simulink model "cbuildv1p1"  (R2024b)
settings: Solver=VariableStepAuto  StartTime=0.0  StopTime=2  RelTol=1e-3
model workspace (MAT data in the model file):
  A_busbar = 0.0015
  A_pack = 0.711626248
  C = 400
  C_nominal = 3
  GR = 14.14
  I_max = 157.708978328
  Izz = 76.97
  P = 5
  P_DD = 1
  REGEN_GAIN = 1
  R_e = 0.197
  S = 138
  SW_TV_GAIN = 0.035
  SoC_initial = 1
  TC_CUT = 0.5
  T_amb = 297.15
  Tmax = 21
  W_max = 34
  a = 0.7497
  busbar_CC_area = 0.000108
  busbar_Cp = 237
  busbar_length = 0.032
  busbar_mass = 0.01
  busbar_resistivity = 1.68e-08
  busbar_thermalcontact_resistance = 1
  c_factor = 0.244
  cell_Cp = 1000
  cell_mass = 0.046
  deg_to_rad = 0.0174533
  g = 9.81
  h_busbar = 5
  h_pack = 5
  kappa_thresh = 0.12
  l = 1.53
  mpersec_to_kph = 3.6
  rackdisp_to_steerangle = 1.29615626969
  rad_to_deg = 57.2958
  rpm_to_radpers = 0.10472
libraries: Solver_SF x1
settings Model: Creator=account  LastModifiedBy=kara.28

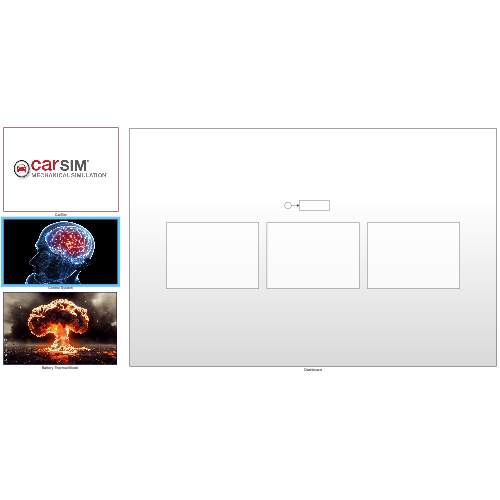
[thumbnail: Simulink's stored preview of the top-level diagram]
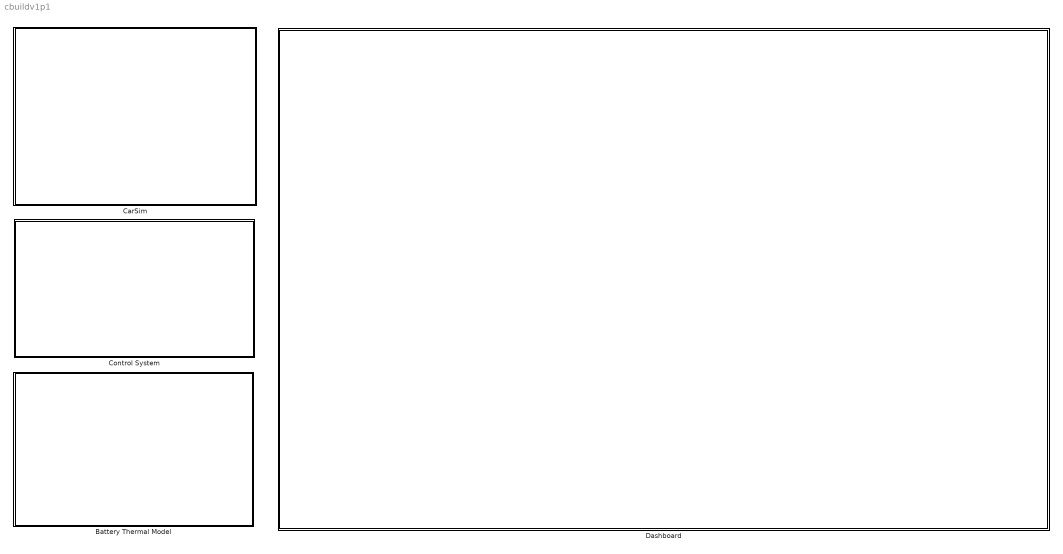
== system cbuildv1p1 ==
  Battery Thermal Model : Subsystem
      mask Display: image('battery.jpg');
  CarSim : Subsystem
      mask Display: image('carsimlogo.jpg');
  Control System : Subsystem
      mask Display: image('controller.jpg');
  Dashboard : Subsystem

== system cbuildv1p1/Battery Thermal Model ==
  Battery Cells : Subsystem
  Busbars : Subsystem

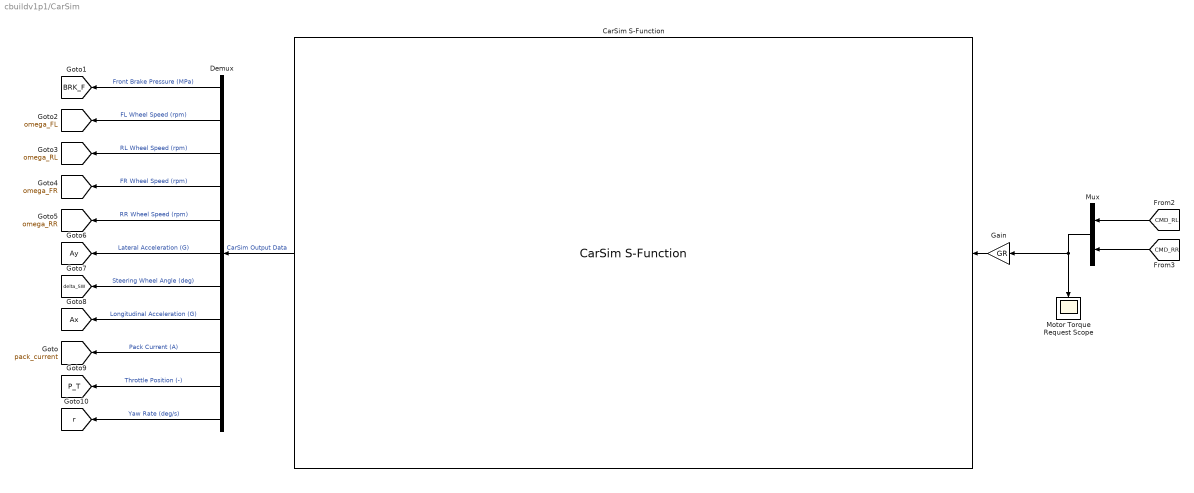
== system cbuildv1p1/CarSim ==
  CarSim S-Function : Solver_SF/CarSim S-Function  Priority=1  SIMFILE=simfile.sim  Run_RTs=off  vs_state_ind=Run  StopMode_ind=Vehicle Model
  Demux : Demux  Outputs=11
  Gain : Gain  Gain=GR
  Motor Torque Request Scope : Scope
  Mux : Mux  Inputs=2
  tag scope: Ax=global, Ay=global, BRK_F=global, P_T=global, delta_SW=global, omega_FL=global, omega_FR=global, omega_RL=global, omega_RR=global, pack_current=global, r=global
  wires:
  Demux/5 -> [omega_RR]  "RR Wheel Speed (rpm)"
  Demux/10 -> [P_T]  "Throttle Position (-)"
  Demux/8 -> [Ax]  "Longitudinal Acceleration (G)"
  Demux/4 -> [omega_FR]  "FR Wheel Speed (rpm)"
  Demux/2 -> [omega_FL]  "FL Wheel Speed (rpm)"
  CarSim S-Function/1 -> Demux/1  "CarSim Output Data"
  Demux/7 -> [delta_SW]  "Steering Wheel Angle (deg)"
  [CMD_RR] -> Mux/2
  [CMD_RL] -> Mux/1
  Demux/9 -> [pack_current]  "Pack Current (A)"
  Demux/3 -> [omega_RL]  "RL Wheel Speed (rpm)"
  Demux/1 -> [BRK_F]  "Front Brake Pressure (MPa)"
  Demux/6 -> [Ay]  "Lateral Acceleration (G)"
  Gain/1 -> CarSim S-Function/1
  Mux/1 -> Gain/1, Motor Torque Request Scope/1
  Demux/11 -> [r]  "Yaw Rate (deg/s)"

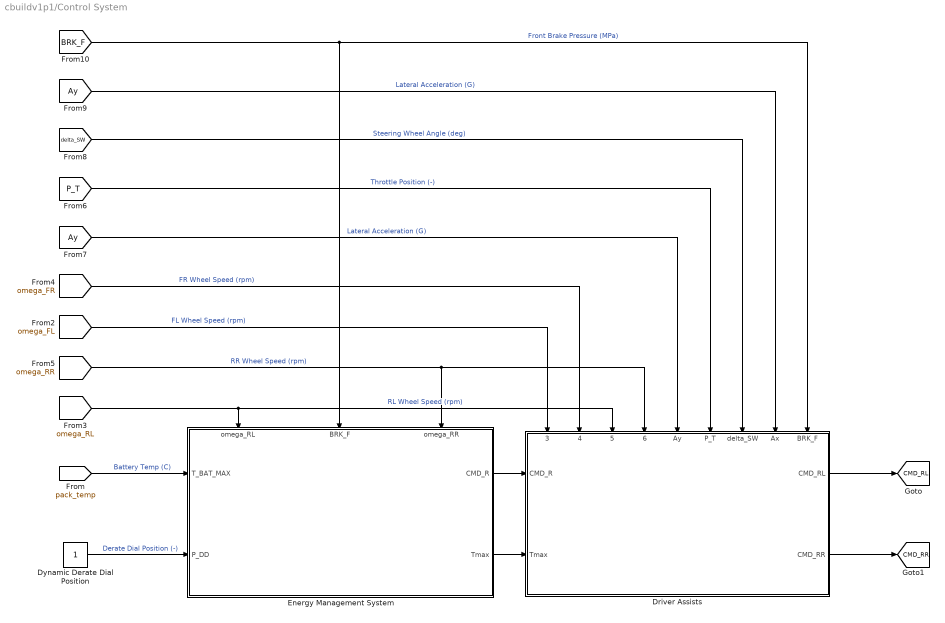
== system cbuildv1p1/Control System ==
  Driver Assists : Subsystem
      settings: PortSchema="{\"entries\":[{\"content\":{\"sides\":[{\"content\":{\"connectorIds\":[\"In1\",\"In2\"]},\"type\":\"ConnectorPlacement.EquallySpacedRectSide\",\"uuid\":\"c30f5bbb-5f7b-4b8f-a220-579b9cc0865f\"},{\"content\":{\"connectorIds\":[\"Out1\",\"Out2\"],\"side\":\"RIGHT\"},\"type\":\"ConnectorPlacement.EquallySpacedRectSide\",\"uuid\":\"8399a92e-19c3-49c4-801c-f7e7f76799cf\"},{\"content\":{\"connectorIds\":[\"In3\",\"In4\",\"In5\",\"In6\",\"In7\",\"In8\",\"In9\",\"In10\",\"In11\"],\"side\":\"TOP\"},\"type\":\"ConnectorPlacement.EquallySpacedRectSide\",\"uuid\":\"19d8375b-8353-4f23-adee-fcd0b0fbd4ef\"}]},\"type\":\"ConnectorPlacement.EquallySpacedConnector\",\"uuid\":\"53834b5a-6686-42bc-a078-9cae71bfd001\"}],\"packageUris\":[\"http://schema.mathworks.com/mf0/Connector/R2020b\"],\"version\":\"1.0\"}"
  Dynamic Derate Dial Position : Constant
  Energy Management System : Subsystem
      settings: PortSchema="{\"entries\":[{\"content\":{\"sides\":[{\"content\":{\"connectorIds\":[\"In1\",\"In2\"]},\"type\":\"ConnectorPlacement.EquallySpacedRectSide\",\"uuid\":\"89c92abe-ca77-4c48-ba79-1fd8447b36ee\"},{\"content\":{\"connectorIds\":[\"Out1\",\"Out2\"],\"side\":\"RIGHT\"},\"type\":\"ConnectorPlacement.EquallySpacedRectSide\",\"uuid\":\"4a58accb-bbe3-490f-b1ea-5257f75ab2ba\"},{\"content\":{\"connectorIds\":[\"In3\",\"In4\",\"In5\"],\"side\":\"TOP\"},\"type\":\"ConnectorPlacement.EquallySpacedRectSide\",\"uuid\":\"b5e96e52-1098-4ccd-9740-b2b10d8cf6b3\"}]},\"type\":\"ConnectorPlacement.EquallySpacedConnector\",\"uuid\":\"06c6d35a-fc7b-4382-b862-8bbe65743431\"}],\"packageUris\":[\"http://schema.mathworks.com/mf0/Connector/R2020b\"],\"version\":\"1.0\"}"
  tag scope: CMD_RL=global, CMD_RR=global
  wires:
  Energy Management System/1(CMD_R) -> Driver Assists/1(CMD_R)
  Energy Management System/2(Tmax) -> Driver Assists/2(Tmax)
  Driver Assists/1(CMD_RL) -> [CMD_RL]
  Driver Assists/2(CMD_RR) -> [CMD_RR]
  [pack_temp] -> Energy Management System/1(T_BAT_MAX)  "Battery Temp (C)"
  Dynamic Derate Dial Position/1 -> Energy Management System/2(P_DD)  "Derate Dial Position (-)"
  [omega_RR] -> Driver Assists/6(omega_RR), Energy Management System/5(omega_RR)  "RR Wheel Speed (rpm)"
  [omega_FR] -> Driver Assists/4(omega_FR)  "FR Wheel Speed (rpm)"
  [omega_RL] -> Driver Assists/5(omega_RL), Energy Management System/3(omega_RL)  "RL Wheel Speed (rpm)"
  [omega_FL] -> Driver Assists/3(omega_FL)  "FL Wheel Speed (rpm)"
  [Ay] -> Driver Assists/7(Ay)  "Lateral Acceleration (G)"
  [P_T] -> Driver Assists/8(P_T)  "Throttle Position (-)"
  [delta_SW] -> Driver Assists/9(delta_SW)  "Steering Wheel Angle (deg)"
  [Ay] -> Driver Assists/10(Ax)  "Lateral Acceleration (G)"
  [BRK_F] -> Energy Management System/4(BRK_F), Driver Assists/11(BRK_F)  "Front Brake Pressure (MPa)"

== system cbuildv1p1/Dashboard ==
  Battery Info : Subsystem
  Clock1 : Clock
  Controls Info : Subsystem
  General Info : Subsystem
  Simulation Time : Display
  wires:
  Clock1/1 -> Simulation Time/1

== system cbuildv1p1/Battery Thermal Model/Battery Cells ==
  Battery Heat : Subsystem
      settings: PortSchema="{\"entries\":[{\"content\":{\"sides\":[{\"content\":{\"connectorIds\":[\"In1\",\"Out1\",\"In2\",\"In3\"]},\"type\":\"ConnectorPlacement.EquallySpacedRectSide\",\"uuid\":\"0f7c0562-63f7-413a-9c65-7d5d0f23ac53\"},{\"content\":{\"side\":\"RIGHT\"},\"type\":\"ConnectorPlacement.EquallySpacedRectSide\",\"uuid\":\"6856fc4a-e601-47fb-aafe-3183d6398fa2\"},{\"content\":{\"side\":\"TOP\"},\"type\":\"ConnectorPlacement.EquallySpacedRectSide\",\"uuid\":\"93500152-ab0c-4e86-a765-8796b82b9cd6\"}]},\"type\":\"ConnectorPlacement.EquallySpacedConnector\",\"uuid\":\"8bef09a8-0835-4033-ba4e-3f5f6277d0ac\"}],\"packageUris\":[\"http://schema.mathworks.com/mf0/Connector/R2020b\"],\"version\":\"1.0\"}"
  Battery Heat Generation : Subsystem
  Busbar - Segment Heat Flow : Subsystem
      settings: PortSchema="{\"entries\":[{\"content\":{\"sides\":[{\"content\":{},\"type\":\"ConnectorPlacement.EquallySpacedRectSide\",\"uuid\":\"839c7b7c-3d90-4543-803d-828e2cd8ee3e\"},{\"content\":{\"connectorIds\":[\"In1\",\"Out1\"],\"side\":\"RIGHT\"},\"type\":\"ConnectorPlacement.EquallySpacedRectSide\",\"uuid\":\"e3492608-3f40-473c-8392-0c925b682872\"},{\"content\":{\"side\":\"TOP\"},\"type\":\"ConnectorPlacement.EquallySpacedRectSide\",\"uuid\":\"8e15337c-e61d-491c-b508-620217c9bb60\"}]},\"type\":\"ConnectorPlacement.EquallySpacedConnector\",\"uuid\":\"03d3ec16-7a24-4203-9805-446eb586226e\"}],\"packageUris\":[\"http://schema.mathworks.com/mf0/Connector/R2020b\"],\"version\":\"1.0\"}"
  Heat Loss : Subsystem
      settings: PortSchema="{\"entries\":[{\"content\":{\"sides\":[{\"content\":{},\"type\":\"ConnectorPlacement.EquallySpacedRectSide\",\"uuid\":\"cd11f8f0-ebc0-4dda-8c98-00f5919de41a\"},{\"content\":{\"connectorIds\":[\"In1\",\"Out1\"],\"side\":\"RIGHT\"},\"type\":\"ConnectorPlacement.EquallySpacedRectSide\",\"uuid\":\"2a68a9a1-bd97-4a17-8a8b-1aa98e9bd9a8\"},{\"content\":{\"side\":\"TOP\"},\"type\":\"ConnectorPlacement.EquallySpacedRectSide\",\"uuid\":\"debcc510-941b-4448-a371-f67c84c59f32\"}]},\"type\":\"ConnectorPlacement.EquallySpacedConnector\",\"uuid\":\"91559e46-754b-48b4-ac3e-ab135f9add0a\"}],\"packageUris\":[\"http://schema.mathworks.com/mf0/Connector/R2020b\"],\"version\":\"1.0\"}"
  Pack Voltage : Subsystem
  wires:
  Battery Heat/1(Pack Temp (K)) -> Busbar - Segment Heat Flow/1(Segment Temp (K)), Heat Loss/1(Pack Temp (K))
  Battery Heat Generation/1(Cell Heat Generation Rate) -> Battery Heat/1(Battery Heat Generation)
  Heat Loss/1(Pack Heat Loss Rate) -> Battery Heat/2(Battery Heat Loss)
  Busbar - Segment Heat Flow/1(Busbar - Segment Heat Flow (W)) -> Battery Heat/3(Busbar - Segment Heat Flow (W))

== system cbuildv1p1/Battery Thermal Model/Busbars ==
  Ambient Heat Loss : Subsystem
      settings: PortSchema="{\"entries\":[{\"content\":{\"sides\":[{\"content\":{},\"type\":\"ConnectorPlacement.EquallySpacedRectSide\",\"uuid\":\"cd11f8f0-ebc0-4dda-8c98-00f5919de41a\"},{\"content\":{\"connectorIds\":[\"In1\",\"Out1\"],\"side\":\"RIGHT\"},\"type\":\"ConnectorPlacement.EquallySpacedRectSide\",\"uuid\":\"2a68a9a1-bd97-4a17-8a8b-1aa98e9bd9a8\"},{\"content\":{\"side\":\"TOP\"},\"type\":\"ConnectorPlacement.EquallySpacedRectSide\",\"uuid\":\"debcc510-941b-4448-a371-f67c84c59f32\"}]},\"type\":\"ConnectorPlacement.EquallySpacedConnector\",\"uuid\":\"91559e46-754b-48b4-ac3e-ab135f9add0a\"}],\"packageUris\":[\"http://schema.mathworks.com/mf0/Connector/R2020b\"],\"version\":\"1.0\"}"
  Busbar - Segment Heat Flow : Subsystem
      settings: PortSchema="{\"entries\":[{\"content\":{\"sides\":[{\"content\":{},\"type\":\"ConnectorPlacement.EquallySpacedRectSide\",\"uuid\":\"839c7b7c-3d90-4543-803d-828e2cd8ee3e\"},{\"content\":{\"connectorIds\":[\"In1\",\"Out1\"],\"side\":\"RIGHT\"},\"type\":\"ConnectorPlacement.EquallySpacedRectSide\",\"uuid\":\"e3492608-3f40-473c-8392-0c925b682872\"},{\"content\":{\"side\":\"TOP\"},\"type\":\"ConnectorPlacement.EquallySpacedRectSide\",\"uuid\":\"8e15337c-e61d-491c-b508-620217c9bb60\"}]},\"type\":\"ConnectorPlacement.EquallySpacedConnector\",\"uuid\":\"03d3ec16-7a24-4203-9805-446eb586226e\"}],\"packageUris\":[\"http://schema.mathworks.com/mf0/Connector/R2020b\"],\"version\":\"1.0\"}"
  Busbar Heat : Subsystem
      settings: PortSchema="{\"entries\":[{\"content\":{\"sides\":[{\"content\":{\"connectorIds\":[\"In1\",\"Out1\",\"In2\",\"In3\"]},\"type\":\"ConnectorPlacement.EquallySpacedRectSide\",\"uuid\":\"0f7c0562-63f7-413a-9c65-7d5d0f23ac53\"},{\"content\":{\"side\":\"RIGHT\"},\"type\":\"ConnectorPlacement.EquallySpacedRectSide\",\"uuid\":\"6856fc4a-e601-47fb-aafe-3183d6398fa2\"},{\"content\":{\"side\":\"TOP\"},\"type\":\"ConnectorPlacement.EquallySpacedRectSide\",\"uuid\":\"93500152-ab0c-4e86-a765-8796b82b9cd6\"}]},\"type\":\"ConnectorPlacement.EquallySpacedConnector\",\"uuid\":\"8bef09a8-0835-4033-ba4e-3f5f6277d0ac\"}],\"packageUris\":[\"http://schema.mathworks.com/mf0/Connector/R2020b\"],\"version\":\"1.0\"}"
  Resistance Heat Generation : Subsystem
  wires:
  Busbar Heat/1(Busbar Temp (K)) -> Busbar - Segment Heat Flow/1(Busbar Temp (K)), Ambient Heat Loss/1(Busbar Temp (K))
  Resistance Heat Generation/1(Busbar Heat Generation Rate) -> Busbar Heat/1(Busbar Heat Generation)
  Ambient Heat Loss/1(Busbar Heat Loss Rate) -> Busbar Heat/2(Busbar Heat Loss)
  Busbar - Segment Heat Flow/1(Busbar - Segment Heat Flow (W)) -> Busbar Heat/3(Busbar - Segment Heat Flow (W))

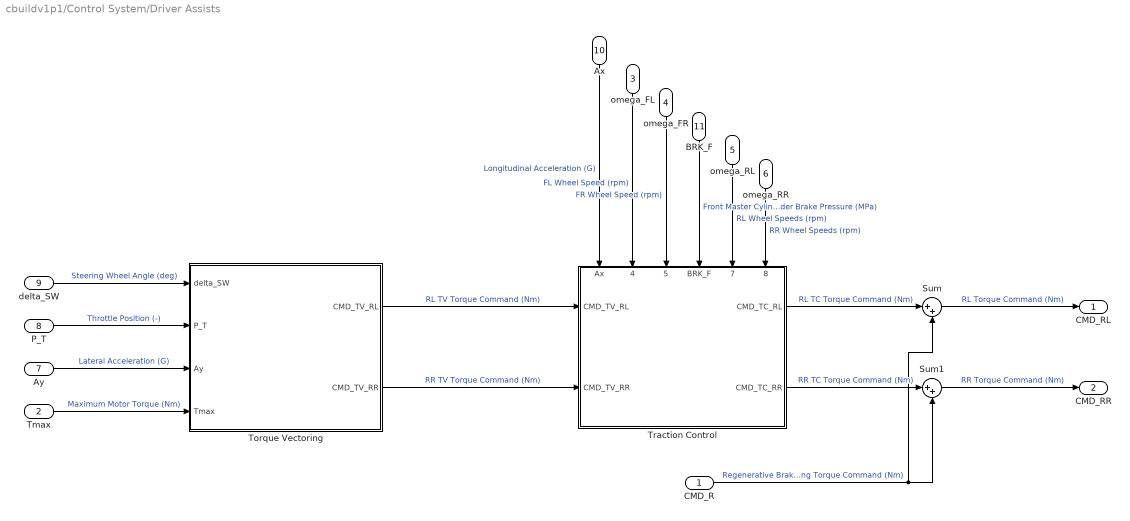
== system cbuildv1p1/Control System/Driver Assists ==
  CMD_R : Inport
  Tmax : Inport  Port=2
  omega_FL : Inport  Port=3
  omega_FR : Inport  Port=4
  omega_RL : Inport  Port=5
  omega_RR : Inport  Port=6
  Ay : Inport  Port=7
  P_T : Inport  Port=8
  delta_SW : Inport  Port=9
  Ax : Inport  Port=10
  BRK_F : Inport  Port=11
  Sum : Sum  Inputs=|++
  Sum1 : Sum  Inputs=|++
  Torque Vectoring : Subsystem
  Traction Control : Subsystem
      settings: PortSchema="{\"entries\":[{\"content\":{\"sides\":[{\"content\":{\"connectorIds\":[\"In1\",\"In2\"]},\"type\":\"ConnectorPlacement.EquallySpacedRectSide\",\"uuid\":\"d61c18bd-9535-4dda-869d-17effaf93de7\"},{\"content\":{\"connectorIds\":[\"Out1\",\"Out2\"],\"side\":\"RIGHT\"},\"type\":\"ConnectorPlacement.EquallySpacedRectSide\",\"uuid\":\"01ce504d-a060-4358-8411-664eedaba102\"},{\"content\":{\"connectorIds\":[\"In3\",\"In4\",\"In5\",\"In6\",\"In7\",\"In8\"],\"side\":\"TOP\"},\"type\":\"ConnectorPlacement.EquallySpacedRectSide\",\"uuid\":\"26eb6c05-86e8-47d0-a1b5-f53131bb5e60\"}]},\"type\":\"ConnectorPlacement.EquallySpacedConnector\",\"uuid\":\"a0cd41b8-03b3-4f62-a25e-73ac641935b2\"}],\"packageUris\":[\"http://schema.mathworks.com/mf0/Connector/R2020b\"],\"version\":\"1.0\"}"
  CMD_RL : Outport
  CMD_RR : Outport  Port=2
  wires:
  Torque Vectoring/2(CMD_TV_RR) -> Traction Control/2(CMD_TV_RR)  "RR TV Torque Command (Nm)"
  delta_SW/1 -> Torque Vectoring/1(delta_SW)  "Steering Wheel Angle (deg)"
  P_T/1 -> Torque Vectoring/2(P_T)  "Throttle Position (-)"
  Ay/1 -> Torque Vectoring/3(Ay)  "Lateral Acceleration (G)"
  Tmax/1 -> Torque Vectoring/4(Tmax)  "Maximum Motor Torque (Nm)"
  Sum/1 -> CMD_RL/1  "RL Torque Command (Nm)"
  Sum1/1 -> CMD_RR/1  "RR Torque Command (Nm)"
  CMD_R/1 -> Sum/2, Sum1/2  "Regenerative Braking Torque Command (Nm)"
  Ax/1 -> Traction Control/3(Ax)  "Longitudinal Acceleration (G)"
  omega_FL/1 -> Traction Control/4(omega_FL)  "FL Wheel Speed (rpm)"
  omega_FR/1 -> Traction Control/5(omega_FR)  "FR Wheel Speed (rpm)"
  BRK_F/1 -> Traction Control/6(BRK_F)  "Front Master Cylinder Brake Pressure (MPa)"
  omega_RL/1 -> Traction Control/7(omega_RL)  "RL Wheel Speeds (rpm)"
  omega_RR/1 -> Traction Control/8(omega_RR)  "RR Wheel Speeds (rpm)"
  Torque Vectoring/1(CMD_TV_RL) -> Traction Control/1(CMD_TV_RL)  "RL TV Torque Command (Nm)"
  Traction Control/1(CMD_TC_RL) -> Sum/1  "RL TC Torque Command (Nm)"
  Traction Control/2(CMD_TC_RR) -> Sum1/1  "RR TC Torque Command (Nm)"

== system cbuildv1p1/Control System/Energy Management System ==
  T_BAT_MAX : Inport
  P_DD : Inport  Port=2
  omega_RL : Inport  Port=3
  BRK_F : Inport  Port=4
  omega_RR : Inport  Port=5
  Dynamic Derate : Subsystem
  Regenerative Braking : Subsystem
  CMD_R : Outport
  Tmax : Outport  Port=2
  wires:
  T_BAT_MAX/1 -> Dynamic Derate/1(T_BAT_MAX)  "Maximum Module Temp (C)"
  P_DD/1 -> Dynamic Derate/2(P_DD)  "Dynamic Derate Dial Position (-)"
  BRK_F/1 -> Regenerative Braking/1(BRK_F)  "Front Master Cylinder Pressure (MPa)"
  Dynamic Derate/1(Tmax) -> Tmax/1  "Maximum Motor Torque (Nm)"
  Regenerative Braking/1(CMD_R) -> CMD_R/1  "Regen Brake Torque Command (Nm)"
  omega_RL/1 -> Dynamic Derate/3(omega_RL)  "RL Wheel Speed (rpm)"
  omega_RR/1 -> Dynamic Derate/4(omega_RR)  "RR Wheel Speed (rpm)"

== system cbuildv1p1/Dashboard/Battery Info ==
  Acceleration Scope : DashboardScope  Ymin=-2.5  Ymax=2.5
  Acceleration Scope1 : DashboardScope  Ymin=0  Ymax=60
  Acceleration Scope2 : DashboardScope  Ymin=0  Ymax=1
  Acceleration Scope3 : DashboardScope  Ymin=0  Ymax=1
  Acceleration Scope4 : DashboardScope  Ymin=0  Ymax=500

== system cbuildv1p1/Dashboard/Controls Info ==
  Acceleration Scope : DashboardScope  Ymin=-2.5  Ymax=2.5
  Acceleration Scope1 : DashboardScope  Ymin=-2  Ymax=2
  Acceleration Scope2 : DashboardScope  Ymin=0  Ymax=1
  Acceleration Scope3 : DashboardScope  Ymin=0  Ymax=80
  Acceleration Scope4 : DashboardScope  Ymin=0  Ymax=21
  Lamp : LampBlock  LabelPosition=Hide
  Rotary Switch : RotarySwitchBlock
      settings: Values={{'DD 1', 'DD 2'}, [0 1]}

== system cbuildv1p1/Dashboard/General Info ==
  Acceleration Scope : DashboardScope  Ymin=-2.5  Ymax=2.5
  Acceleration Scope1 : DashboardScope  Ymin=0  Ymax=110
  Acceleration Scope2 : DashboardScope  Ymin=0  Ymax=1
  Acceleration Scope3 : DashboardScope  Ymin=0  Ymax=10
  Acceleration Scope4 : DashboardScope  Ymin=0  Ymax=150

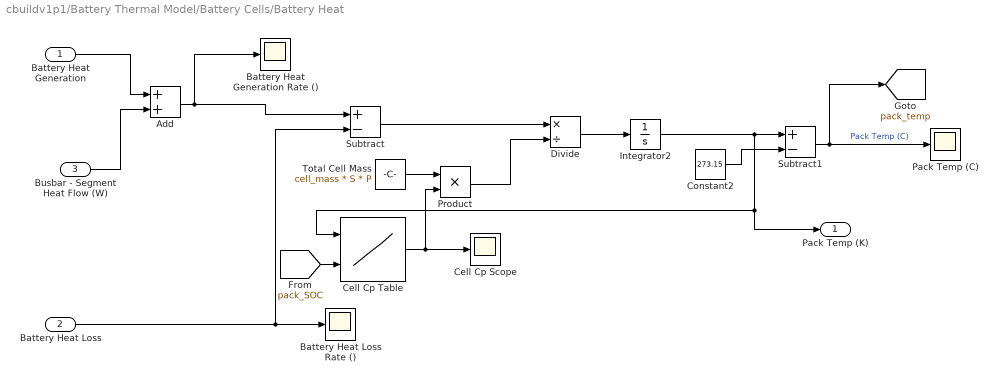
== system cbuildv1p1/Battery Thermal Model/Battery Cells/Battery Heat ==
  Battery Heat Generation : Inport
  Battery Heat Loss : Inport  Port=2
  Busbar - Segment Heat Flow (W) : Inport  Port=3
  Add : Sum
  Battery Heat Generation Rate () : Scope
  Battery Heat Loss Rate () : Scope
  Cell Cp Scope : Scope
  Cell Cp Table : Lookup_n-D  BreakpointsForDimension1=[296.0488;303.3425;312.147;321.5769;330.6423]  BreakpointsForDimension2=[0 0.5 1]  Table=[811.0868 819.6535 830.8545;814.1373 822.704 834.6964;817.9826 826.8129 838.6737000000001;822.2249 831.0552 843.4446;826.7299 835.8239 848.3459]  InterpMethod=Cubic spline  InternalRulePriority=Speed  RndMeth=Simplest
      settings: InputPortMap=u0,u1
  Constant2 : Constant  Value=273.15
  Divide : Product  Inputs=*/
  Integrator2 : Integrator  InitialCondition=T_amb
  Pack Temp (C) : Scope
  Product : Product
  Subtract : Sum  Inputs=+-
  Subtract1 : Sum  Inputs=+-
  Total Cell Mass : Constant  Value=cell_mass * S * P
  Pack Temp (K) : Outport
  tag scope: pack_temp=global
  wires:
  Cell Cp Table/1 -> Product/2, Cell Cp Scope/1
  Constant2/1 -> Subtract1/2
  Divide/1 -> Integrator2/1
  Subtract/1 -> Divide/1
  Integrator2/1 -> Pack Temp (K)/1, Cell Cp Table/1, Subtract1/1
  Subtract1/1 -> [pack_temp], Pack Temp (C)/1  "Pack Temp (C)"
  Total Cell Mass/1 -> Product/1
  Product/1 -> Divide/2
  Battery Heat Loss/1 -> Battery Heat Loss Rate ()/1, Subtract/2
  Battery Heat Generation/1 -> Add/1
  Busbar - Segment Heat Flow (W)/1 -> Add/2
  Add/1 -> Subtract/1, Battery Heat Generation Rate ()/1
  [pack_SOC] -> Cell Cp Table/2

== system cbuildv1p1/Battery Thermal Model/Battery Cells/Battery Heat Generation ==
  Cell Resistance : Subsystem
      settings: PortSchema="{\"entries\":[{\"content\":{\"sides\":[{\"content\":{},\"type\":\"ConnectorPlacement.EquallySpacedRectSide\",\"uuid\":\"1c6ff2a8-2c86-4b92-aa7d-5717a02d6f28\"},{\"content\":{\"connectorIds\":[\"In1\",\"In2\",\"Out1\"],\"side\":\"RIGHT\"},\"type\":\"ConnectorPlacement.EquallySpacedRectSide\",\"uuid\":\"52a4cb2c-e1db-459d-bd0a-206cc3bba6d1\"},{\"content\":{\"side\":\"TOP\"},\"type\":\"ConnectorPlacement.EquallySpacedRectSide\",\"uuid\":\"751bbbd6-abc7-4265-8d68-4aa70d69379f\"}]},\"type\":\"ConnectorPlacement.EquallySpacedConnector\",\"uuid\":\"b8f9630f-0167-4478-8d98-637e13782dcd\"}],\"packageUris\":[\"http://schema.mathworks.com/mf0/Connector/R2020b\"],\"version\":\"1.0\"}"
  Cells in Parallel : Constant  Value=P
  Cells in series : Constant  Value=S
  Current Estimator : Subsystem
  Divide : Product  Inputs=*/
  Pack SoC : Subsystem
      settings: PortSchema="{\"entries\":[{\"content\":{\"sides\":[{\"content\":{},\"type\":\"ConnectorPlacement.EquallySpacedRectSide\",\"uuid\":\"1c6ff2a8-2c86-4b92-aa7d-5717a02d6f28\"},{\"content\":{\"connectorIds\":[\"In1\",\"Out1\"],\"side\":\"RIGHT\"},\"type\":\"ConnectorPlacement.EquallySpacedRectSide\",\"uuid\":\"52a4cb2c-e1db-459d-bd0a-206cc3bba6d1\"},{\"content\":{\"side\":\"TOP\"},\"type\":\"ConnectorPlacement.EquallySpacedRectSide\",\"uuid\":\"751bbbd6-abc7-4265-8d68-4aa70d69379f\"}]},\"type\":\"ConnectorPlacement.EquallySpacedConnector\",\"uuid\":\"b8f9630f-0167-4478-8d98-637e13782dcd\"}],\"packageUris\":[\"http://schema.mathworks.com/mf0/Connector/R2020b\"],\"version\":\"1.0\"}"
  Product : Product
  Product1 : Product
  Product2 : Product
  Square : Math  Operator=square
  Cell Heat Generation Rate : Outport
  wires:
  Cells in series/1 -> Product1/1
  Divide/1 -> Cell Resistance/1(Cell Current  (A)), Square/1  "Cell Current (A)"
  Cell Resistance/1(Cell Resistance (ohms)) -> Product/2  "Cell Resistance (ohms)"
  Square/1 -> Product/1
  Cells in Parallel/1 -> Divide/2, Product1/2
  Product1/1 -> Product2/2
  Product/1 -> Product2/1  "Pack Heat Generation Rate (W)"
  Product2/1 -> Cell Heat Generation Rate/1  "Cell Heat Generation Rate (W)"
  Pack SoC/1(SoC (%)) -> Cell Resistance/2(SoC (%))  "Pack SoC (-)"
  Current Estimator/1(Pack Current (A)) -> Pack SoC/1(Pack Current (A)), Divide/1  "Pack Current (A)"

== system cbuildv1p1/Battery Thermal Model/Battery Cells/Busbar - Segment Heat Flow ==
  Segment Temp (K) : Inport
  Add : Sum
  Constant : Constant  Value=busbar_thermalcontact_resistance
  Constant1 : Constant  Value=273.15
  Divide : Product  Inputs=*/
  Subtract : Sum  Inputs=+-
  Busbar - Segment Heat Flow (W) : Outport
  wires:
  Subtract/1 -> Divide/1  "Temp diff (K)"
  Constant/1 -> Divide/2
  Divide/1 -> Busbar - Segment Heat Flow (W)/1
  [busbar_temp] -> Add/2  "Segment temp (C)"
  Constant1/1 -> Add/1
  Segment Temp (K)/1 -> Subtract/1
  Add/1 -> Subtract/2  "Segment temp (K)"

== system cbuildv1p1/Battery Thermal Model/Battery Cells/Heat Loss ==
  Pack Temp (K) : Inport
  Constant : Constant  Value=h_pack
  Constant1 : Constant  Value=T_amb
  Gain : Gain  Gain=A_pack
  Product : Product
  Scope : Scope
  Subtract : Sum  Inputs=+-
  Pack Heat Loss Rate : Outport
  tag scope: pack_heatloss=global
  wires:
  Constant/1 -> Gain/1
  Subtract/1 -> Product/2, Scope/1
  Gain/1 -> Product/1
  Product/1 -> [pack_heatloss], Pack Heat Loss Rate/1
  Pack Temp (K)/1 -> Subtract/1
  Constant1/1 -> Subtract/2

== system cbuildv1p1/Battery Thermal Model/Battery Cells/Pack Voltage ==
  Gain : Gain  Gain=S
  Lookup with Linear Lagrange Interpolation : Lookup_n-D  NumberOfTableDimensions=1  BreakpointsForDimension1=[0.100961;0.201247;0.30155;0.401865;0.502237;0.602602;0.7029339999999999;0.8032629999999999;0.903617;1]  Table=[3.227877;3.437376;3.537935;3.663634;3.755814;3.835423;3.940172;4.047017;4.097296;4.187904]  InterpMethod=Cubic spline  InternalRulePriority=Speed  RndMeth=Simplest
  tag scope: pack_OCV=global
  wires:
  [pack_SOC] -> Lookup with Linear Lagrange Interpolation/1
  Lookup with Linear Lagrange Interpolation/1 -> Gain/1
  Gain/1 -> [pack_OCV]  "Pack OCV (V)"

== system cbuildv1p1/Battery Thermal Model/Busbars/Ambient Heat Loss ==
  Busbar Temp (K) : Inport
  Ambient temp (K) : Constant  Value=T_amb
  H busbar : Constant  Value=h_busbar
  Product : Product
  Subtract : Sum  Inputs=+-
  busbar area : Gain  Gain=A_busbar
  Busbar Heat Loss Rate : Outport
  tag scope: busbar_heatloss=global
  wires:
  H busbar/1 -> busbar area/1
  Subtract/1 -> Product/2
  busbar area/1 -> Product/1
  Product/1 -> [busbar_heatloss], Busbar Heat Loss Rate/1
  Busbar Temp (K)/1 -> Subtract/1
  Ambient temp (K)/1 -> Subtract/2

== system cbuildv1p1/Battery Thermal Model/Busbars/Busbar - Segment Heat Flow ==
  Busbar Temp (K) : Inport
  Add : Sum
  Constant : Constant  Value=busbar_thermalcontact_resistance
  Constant1 : Constant  Value=273.15
  Divide : Product  Inputs=*/
  Subtract : Sum  Inputs=+-
  Busbar - Segment Heat Flow (W) : Outport
  tag scope: busbar_segment_heatflow=global
  wires:
  Busbar Temp (K)/1 -> Subtract/2
  Subtract/1 -> Divide/1  "Temp diff (K)"
  Constant/1 -> Divide/2
  Divide/1 -> [busbar_segment_heatflow], Busbar - Segment Heat Flow (W)/1
  [pack_temp] -> Add/2  "Segment temp (C)"
  Constant1/1 -> Add/1
  Add/1 -> Subtract/1  "Segment temp (K)"

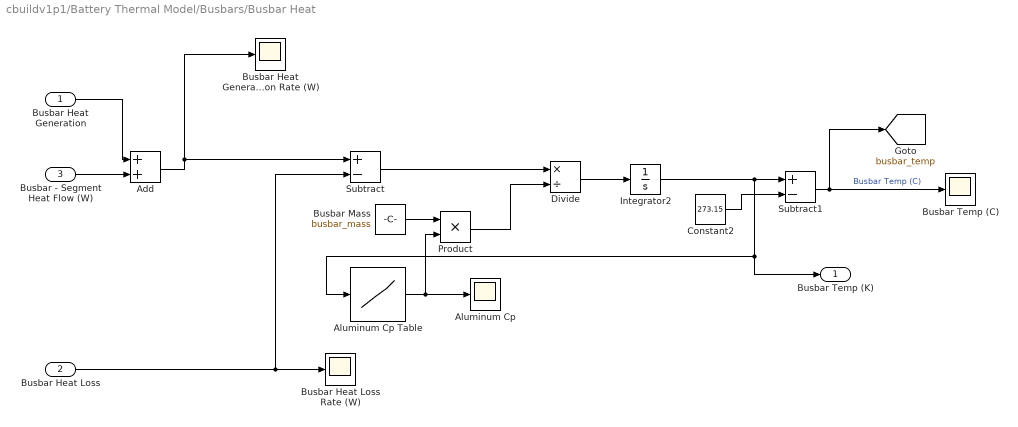
== system cbuildv1p1/Battery Thermal Model/Busbars/Busbar Heat ==
  Busbar Heat Generation : Inport
  Busbar Heat Loss : Inport  Port=2
  Busbar - Segment Heat Flow (W) : Inport  Port=3
  Add : Sum
  Aluminum Cp : Scope
  Aluminum Cp Table : Lookup_n-D  NumberOfTableDimensions=1  BreakpointsForDimension1=[298;300;400;500;600;700;800;900]  Table=[380.7;381.6;405.6;422.3;438.8;457.9;480.9;508.3]  InterpMethod=Cubic spline  InternalRulePriority=Speed  RndMeth=Simplest
  Busbar Heat Generation Rate (W) : Scope
  Busbar Heat Loss Rate (W) : Scope
  Busbar Mass : Constant  Value=busbar_mass
  Busbar Temp (C) : Scope
  Constant2 : Constant  Value=273.15
  Divide : Product  Inputs=*/
  Integrator2 : Integrator  InitialCondition=T_amb
  Product : Product
  Subtract : Sum  Inputs=+-
  Subtract1 : Sum  Inputs=+-
  Busbar Temp (K) : Outport
  tag scope: busbar_temp=global
  wires:
  Aluminum Cp Table/1 -> Product/2, Aluminum Cp/1
  Constant2/1 -> Subtract1/2
  Busbar Heat Generation/1 -> Add/1
  Divide/1 -> Integrator2/1
  Subtract/1 -> Divide/1
  Integrator2/1 -> Aluminum Cp Table/1, Busbar Temp (K)/1, Subtract1/1
  Subtract1/1 -> [busbar_temp], Busbar Temp (C)/1  "Busbar Temp (C)"
  Busbar Mass/1 -> Product/1
  Product/1 -> Divide/2
  Busbar Heat Loss/1 -> Busbar Heat Loss Rate (W)/1, Subtract/2
  Busbar - Segment Heat Flow (W)/1 -> Add/2
  Add/1 -> Subtract/1, Busbar Heat Generation Rate (W)/1

== system cbuildv1p1/Battery Thermal Model/Busbars/Resistance Heat Generation ==
  Busbar cross sectional area (m^2) : Constant  Value=busbar_CC_area
  Busbar length (m) : Constant  Value=busbar_length
  Busbar resistivity (Ohms * m) : Constant  Value=busbar_resistivity
  Divide : Product  Inputs=*/
  Product : Product
  Product1 : Product
  Square : Math  Operator=square
  Busbar Heat Generation Rate : Outport
  wires:
  Product/1 -> Busbar Heat Generation Rate/1  "Busbar Heat Loss (W)"
  [pack_current] -> Square/1  "Pack Current (A)"
  Square/1 -> Product/1
  Busbar resistivity (Ohms * m)/1 -> Product1/1
  Busbar length (m)/1 -> Product1/2
  Product1/1 -> Divide/1
  Busbar cross sectional area (m^2)/1 -> Divide/2
  Divide/1 -> Product/2  "Busbar resistance (ohms)"

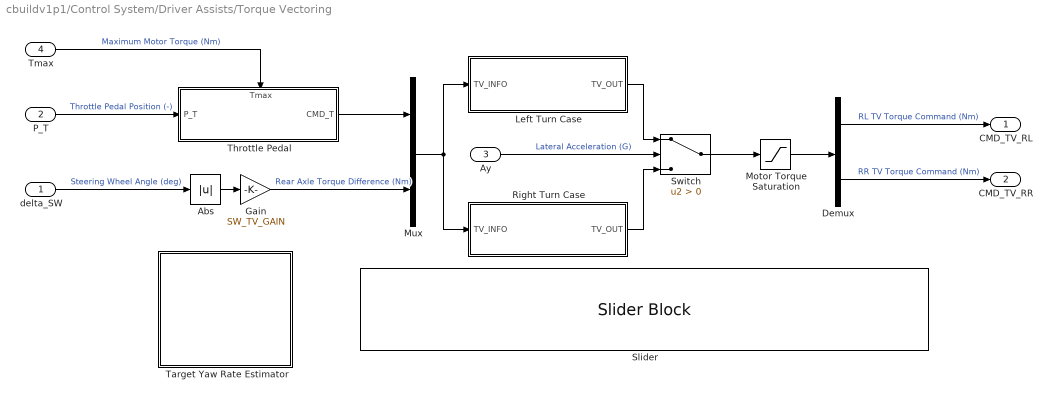
== system cbuildv1p1/Control System/Driver Assists/Torque Vectoring ==
  delta_SW : Inport
  P_T : Inport  Port=2
  Ay : Inport  Port=3
  Tmax : Inport  Port=4
  Abs : Abs  SaturateOnIntegerOverflow=off
  Demux : Demux  Outputs=2
  Gain : Gain  Gain=SW_TV_GAIN
  Left Turn Case : Subsystem
  Motor Torque Saturation : Saturate  UpperLimit=Tmax  LowerLimit=0
  Mux : Mux  Inputs=2
  Right Turn Case : Subsystem
  Slider : SliderBlock  ScaleMax=0.2  TickInterval=0.01
  Switch : Switch  Criteria=u2 > Threshold  SaturateOnIntegerOverflow=off  InputSameDT=off
  Target Yaw Rate Estimator : Subsystem
  Throttle Pedal : Subsystem
      settings: PortSchema="{\"entries\":[{\"content\":{\"sides\":[{\"content\":{\"connectorIds\":[\"In1\"]},\"type\":\"ConnectorPlacement.EquallySpacedRectSide\",\"uuid\":\"2b27b7ae-a1b0-424c-ba89-4fa8e2fb9573\"},{\"content\":{\"connectorIds\":[\"Out1\"],\"side\":\"RIGHT\"},\"type\":\"ConnectorPlacement.EquallySpacedRectSide\",\"uuid\":\"35debb5b-e82d-4475-8dc9-1b915a5a0cae\"},{\"content\":{\"connectorIds\":[\"In2\"],\"side\":\"TOP\"},\"type\":\"ConnectorPlacement.EquallySpacedRectSide\",\"uuid\":\"f3fd2101-c365-4f42-b396-02e014a928b2\"}]},\"type\":\"ConnectorPlacement.EquallySpacedConnector\",\"uuid\":\"f19feaaa-e3f7-4392-8847-f37ac3c71c65\"}],\"packageUris\":[\"http://schema.mathworks.com/mf0/Connector/R2020b\"],\"version\":\"1.0\"}"
  CMD_TV_RL : Outport
  CMD_TV_RR : Outport  Port=2
  wires:
  delta_SW/1 -> Abs/1  "Steering Wheel Angle (deg)"
  P_T/1 -> Throttle Pedal/1(P_T)  "Throttle Pedal Position (-)"
  Ay/1 -> Switch/2  "Lateral Acceleration (G)"
  Mux/1 -> Right Turn Case/1(TV_INFO), Left Turn Case/1(TV_INFO)
  Throttle Pedal/1(CMD_T) -> Mux/1
  Gain/1 -> Mux/2  "Rear Axle Torque Difference (Nm)"
  Switch/1 -> Motor Torque Saturation/1
  Demux/1 -> CMD_TV_RL/1  "RL TV Torque Command (Nm)"
  Demux/2 -> CMD_TV_RR/1  "RR TV Torque Command (Nm)"
  Left Turn Case/1(TV_OUT) -> Switch/1
  Right Turn Case/1(TV_OUT) -> Switch/3
  Motor Torque Saturation/1 -> Demux/1
  Tmax/1 -> Throttle Pedal/2(Tmax)  "Maximum Motor Torque (Nm)"
  Abs/1 -> Gain/1

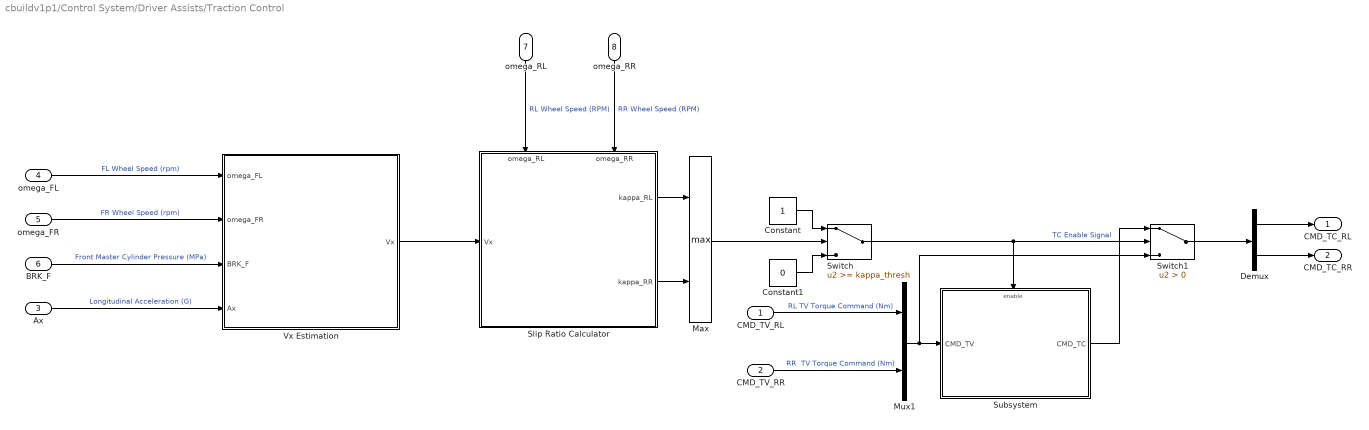
== system cbuildv1p1/Control System/Driver Assists/Traction Control ==
  CMD_TV_RL : Inport
  CMD_TV_RR : Inport  Port=2
  Ax : Inport  Port=3
  omega_FL : Inport  Port=4
  omega_FR : Inport  Port=5
  BRK_F : Inport  Port=6
  omega_RL : Inport  Port=7
  omega_RR : Inport  Port=8
  Constant : Constant
  Constant1 : Constant  Value=0
  Demux : Demux  Outputs=2
  Max : MinMax  Function=max  Inputs=2
  Mux1 : Mux  Inputs=2
  Slip Ratio Calculator : Subsystem
      settings: PortSchema="{\"entries\":[{\"content\":{\"sides\":[{\"content\":{\"connectorIds\":[\"In1\"]},\"type\":\"ConnectorPlacement.EquallySpacedRectSide\",\"uuid\":\"7fdfdad2-33dd-4f06-b604-3c6d01a9d7f8\"},{\"content\":{\"connectorIds\":[\"Out1\",\"Out2\"],\"side\":\"RIGHT\"},\"type\":\"ConnectorPlacement.EquallySpacedRectSide\",\"uuid\":\"dd7c3b4e-ee50-4427-819e-6ce97aa41bd4\"},{\"content\":{\"connectorIds\":[\"In2\",\"In3\"],\"side\":\"TOP\"},\"type\":\"ConnectorPlacement.EquallySpacedRectSide\",\"uuid\":\"78cf20ba-e7fd-4300-9f66-06aa85c1fb42\"}]},\"type\":\"ConnectorPlacement.EquallySpacedConnector\",\"uuid\":\"f81e5908-a010-4627-83b7-5417b93ce453\"}],\"packageUris\":[\"http://schema.mathworks.com/mf0/Connector/R2020b\"],\"version\":\"1.0\"}"
  Subsystem : Subsystem
  Switch : Switch  Threshold=kappa_thresh  SaturateOnIntegerOverflow=off  InputSameDT=off
  Switch1 : Switch  Criteria=u2 > Threshold  SaturateOnIntegerOverflow=off  InputSameDT=off
  Vx Estimation : Subsystem
  CMD_TC_RL : Outport
  CMD_TC_RR : Outport  Port=2
  wires:
  Ax/1 -> Vx Estimation/4(Ax)  "Longitudinal Acceleration (G)"
  omega_FL/1 -> Vx Estimation/1(omega_FL)  "FL Wheel Speed (rpm)"
  omega_FR/1 -> Vx Estimation/2(omega_FR)  "FR Wheel Speed (rpm)"
  BRK_F/1 -> Vx Estimation/3(BRK_F)  "Front Master Cylinder Pressure (MPa)"
  omega_RL/1 -> Slip Ratio Calculator/2(omega_RL)  "RL Wheel Speed (RPM)"
  omega_RR/1 -> Slip Ratio Calculator/3(omega_RR)  "RR Wheel Speed (RPM)"
  Vx Estimation/1(Vx) -> Slip Ratio Calculator/1(Vx)
  Slip Ratio Calculator/1(kappa_RL) -> Max/1
  Slip Ratio Calculator/2(kappa_RR) -> Max/2
  Max/1 -> Switch/2
  Constant/1 -> Switch/1
  Constant1/1 -> Switch/3
  Switch/1 -> Switch1/2, Subsystem/Enable  "TC Enable Signal"
  Subsystem/1(CMD_TC) -> Switch1/1
  CMD_TV_RL/1 -> Mux1/1  "RL TV Torque Command (Nm)"
  CMD_TV_RR/1 -> Mux1/2  "RR  TV Torque Command (Nm)"
  Mux1/1 -> Switch1/3, Subsystem/1(CMD_TV)
  Switch1/1 -> Demux/1
  Demux/1 -> CMD_TC_RL/1
  Demux/2 -> CMD_TC_RR/1

== system cbuildv1p1/Control System/Energy Management System/Dynamic Derate ==
  T_BAT_MAX : Inport
  P_DD : Inport  Port=2
  omega_RL : Inport  Port=3
  omega_RR : Inport  Port=4
  Dynamic Derate 3D LUT : Lookup_n-D  NumberOfTableDimensions=3  BreakpointsForDimension1=[0;25;50;75;100]  BreakpointsForDimension2=[30;50;60;80]  BreakpointsForDimension3=[1 2 3 4]  Table=reshape([73.5 73.5 73.5 73.5 73.5 73.5 73.5 73.5 73.5 73.5 73.5 73.5 73.5 73.5 73.5 73.5 73.5 73.5 73.5 73.5 73.5 73.5 73.5 73.5 73.5 60 60 50 40 30 40 40 30 20 15 20 15 12.5 10 10 36.75 36.75 36.75 36.75 36.75 30 30 25 20 15 20 20 15 10 7.5 10 7.5 6.25 5 5 18.375 18.375 18.375 18.375 18.375 15 15 12.5 10 7.5 10 10 7.5 5 3.75 5 3.75 3.125 2.5 2.5], [5 4 4])  ExtrapMethod=Clip  InternalRulePriority=Speed  RndMeth=Simplest
      settings: InputPortMap=u0,u1,u2
  Gain : Gain  Gain=mpersec_to_kph
  Motor Output Saturation : Saturate  UpperLimit=Tmax  LowerLimit=0
  Motor Torque Calculator : Subsystem
      settings: PortSchema="{\"entries\":[{\"content\":{\"sides\":[{\"content\":{\"connectorIds\":[\"In1\",\"In2\"]},\"type\":\"ConnectorPlacement.EquallySpacedRectSide\",\"uuid\":\"904eb794-76c4-4372-ae2c-4ef2e0000433\"},{\"content\":{\"connectorIds\":[\"Out1\"],\"side\":\"RIGHT\"},\"type\":\"ConnectorPlacement.EquallySpacedRectSide\",\"uuid\":\"8161fba4-68b1-4b44-95f9-b05533d0f86a\"},{\"content\":{\"connectorIds\":[\"In3\"],\"side\":\"TOP\"},\"type\":\"ConnectorPlacement.EquallySpacedRectSide\",\"uuid\":\"e37aa600-3bd6-4b73-8bba-520f94d37a3f\"}]},\"type\":\"ConnectorPlacement.EquallySpacedConnector\",\"uuid\":\"d8616461-ce1c-4b50-a881-919f614525dd\"}],\"packageUris\":[\"http://schema.mathworks.com/mf0/Connector/R2020b\"],\"version\":\"1.0\"}"
  Scope : Scope
  Tmax : Outport
  wires:
  T_BAT_MAX/1 -> Dynamic Derate 3D LUT/1  "Maximum Module Temp (C)"
  [Vx] -> Gain/1
  P_DD/1 -> Dynamic Derate 3D LUT/3  "Dynamic Derate Dial Position (-)"
  Dynamic Derate 3D LUT/1 -> Motor Torque Calculator/3(B_MAX)  "Maximum Battery Power (KW)"
  omega_RL/1 -> Motor Torque Calculator/1(omega_RL)  "RL Wheel Speed (rpm)"
  omega_RR/1 -> Motor Torque Calculator/2(omega_RR)  "RR Wheel Speed (rpm)"
  Motor Torque Calculator/1(Tmax) -> Motor Output Saturation/1  "Maximum Motor Output Torque (Nm)"
  Motor Output Saturation/1 -> Scope/1, Tmax/1
  Gain/1 -> Dynamic Derate 3D LUT/2  "Vehicle Velocity (kph)"

== system cbuildv1p1/Control System/Energy Management System/Regenerative Braking ==
  BRK_F : Inport
  Regen Brake Torque Gain : Gain  Gain=REGEN_GAIN
  CMD_R : Outport
  wires:
  BRK_F/1 -> Regen Brake Torque Gain/1  "Front Master Cylinder Pressure (MPa)"
  Regen Brake Torque Gain/1 -> CMD_R/1  "Regen Brake Torque Command (Nm)"

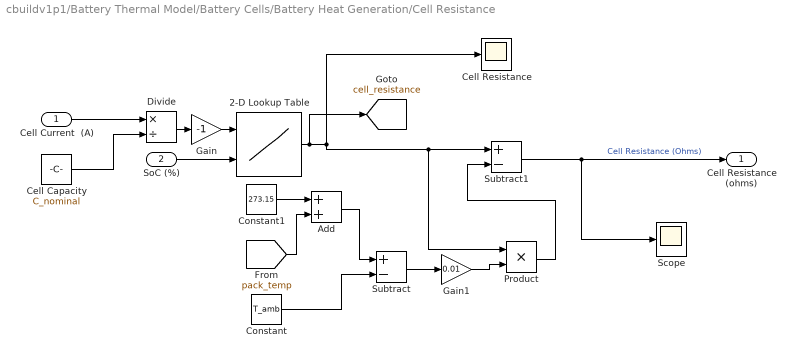
== system cbuildv1p1/Battery Thermal Model/Battery Cells/Battery Heat Generation/Cell Resistance ==
  Cell Current  (A) : Inport
  SoC (%) : Inport  Port=2
  2-D Lookup Table : Lookup_n-D  BreakpointsForDimension1=[-10;-5;-1;1;2;3]  BreakpointsForDimension2=[0.1;0.2;0.3;0.4;0.5;0.6;0.7;0.8;0.9;1]  Table=[0.018906 0.01868 0.018453 0.018226 0.017999 0.017916 0.017743 0.018183 0.019549 0.022703;0.021356 0.020344 0.019332 0.019017 0.018694 0.018598 0.018319 0.018773 0.020642 0.024917;0.02305 0.020909 0.018859 0.019644 0.019687 0.018989 0.018291 0.019295 0.021608 0.026536;0.023001 0.020599 0.019683 0.019161 0.01894 0.018506 0.018636 0.019336 0.020993 0.02265;0.022654 0.020712 0.018901 0.018682 0.018442 0.018289 0.017788 0.017286 0.016785 0.016283;0.019898 0.017891 0.017366 0.01725 0.01725 0.017251 0.017251 0.017251 0.017251 0.017251]  InterpMethod=Cubic spline  ExtrapMethod=Clip  InternalRulePriority=Speed  RndMeth=Simplest
      settings: InputPortMap=u0,u1
  Add : Sum
  Cell Capacity : Constant  Value=C_nominal
  "Cell Resistance " : Scope
  Constant : Constant  Value=T_amb
  Constant1 : Constant  Value=273.15
  Divide : Product  Inputs=*/
  Gain : Gain  Gain=-1
  Gain1 : Gain  Gain=0.01
  Product : Product
  Scope : Scope
  Subtract : Sum  Inputs=+-
  Subtract1 : Sum  Inputs=+-
  Cell Resistance (ohms) : Outport
  tag scope: cell_resistance=global
  wires:
  Cell Current  (A)/1 -> Divide/1
  Cell Capacity/1 -> Divide/2
  SoC (%)/1 -> 2-D Lookup Table/2
  2-D Lookup Table/1 -> Product/1, Subtract1/1, "Cell Resistance "/1, [cell_resistance]
  Divide/1 -> Gain/1
  Gain/1 -> 2-D Lookup Table/1
  Subtract/1 -> Gain1/1
  Constant/1 -> Subtract/2
  [pack_temp] -> Add/2
  Add/1 -> Subtract/1
  Constant1/1 -> Add/1
  Gain1/1 -> Product/2
  Product/1 -> Subtract1/2
  Subtract1/1 -> Cell Resistance (ohms)/1, Scope/1  "Cell Resistance (Ohms)"

== system cbuildv1p1/Battery Thermal Model/Battery Cells/Battery Heat Generation/Current Estimator ==
  Divide : Product  Inputs=*/
  Power Estimator : Subsystem
  Pack Current (A) : Outport
  wires:
  Power Estimator/1(Motor Power (W)) -> Divide/1  "Motor Power (W)"
  Divide/1 -> Pack Current (A)/1  "Pack Current (A)"
  [pack_OCV] -> Divide/2  "Pack Open Circuit Voltage (V)"

== system cbuildv1p1/Battery Thermal Model/Battery Cells/Battery Heat Generation/Pack SoC ==
  Pack Current (A) : Inport
  Constant : Constant  Value=SoC_initial
  Constant1 : Constant  Value=P
  Divide : Product  Inputs=*/
  Gain : Gain  Gain=1/3600
  Integrator : Integrator
  Multiply : Gain  Gain=C_nominal
  Subtract : Sum  Inputs=+-
  SoC (%) : Outport
  tag scope: pack_SOC=global
  wires:
  Pack Current (A)/1 -> Integrator/1
  Constant/1 -> Subtract/1
  Integrator/1 -> Divide/1
  Subtract/1 -> [pack_SOC], SoC (%)/1  "SoC (%)"
  Constant1/1 -> Multiply/1
  Multiply/1 -> Divide/2
  Divide/1 -> Gain/1
  Gain/1 -> Subtract/2

== system cbuildv1p1/Control System/Driver Assists/Torque Vectoring/Left Turn Case ==
  TV_INFO : Inport
  Demux : Demux  Outputs=2
  Mux : Mux  Inputs=2
  Sum : Sum  Inputs=|+-
  Sum1 : Sum  Inputs=|++
  TV_OUT : Outport
  wires:
  TV_INFO/1 -> Demux/1
  Demux/1 -> Sum1/1, Sum/1
  Sum/1 -> Mux/1  "RL TV Torque Command (Nm)"
  Demux/2 -> Sum1/2, Sum/2
  Sum1/1 -> Mux/2  "RR TV Torque Command"
  Mux/1 -> TV_OUT/1

== system cbuildv1p1/Control System/Driver Assists/Torque Vectoring/Right Turn Case ==
  TV_INFO : Inport
  Demux : Demux  Outputs=2
  Mux : Mux  Inputs=2
  Sum : Sum  Inputs=|++
  Sum1 : Sum  Inputs=|+-
  TV_OUT : Outport
  wires:
  Mux/1 -> TV_OUT/1
  Sum/1 -> Mux/1  "RL TV Torque Command (Nm)"
  Demux/2 -> Sum1/2, Sum/2
  Sum1/1 -> Mux/2  "RR TV Torque Command"
  Demux/1 -> Sum1/1, Sum/1
  TV_INFO/1 -> Demux/1

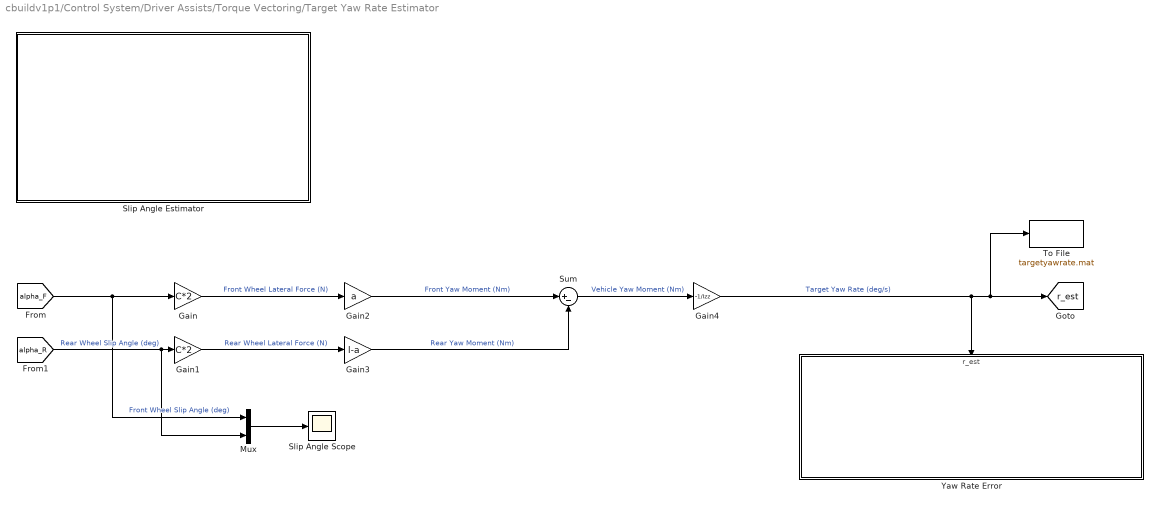
== system cbuildv1p1/Control System/Driver Assists/Torque Vectoring/Target Yaw Rate Estimator ==
  Gain : Gain  Gain=C*2
  Gain1 : Gain  Gain=C*2
  Gain2 : Gain  Gain=a
  Gain3 : Gain  Gain=l-a
  Gain4 : Gain  Gain=-1/Izz
  Mux : Mux  Inputs=2
  Slip Angle Estimator : Subsystem
  Slip Angle Scope : Scope
  Sum : Sum  Inputs=|+-
  To File : ToFile  Filename=targetyawrate.mat
  Yaw Rate Error : Subsystem
      settings: PortSchema="{\"entries\":[{\"content\":{\"sides\":[{\"content\":{},\"type\":\"ConnectorPlacement.EquallySpacedRectSide\",\"uuid\":\"b231141e-075c-44c2-9b61-2a7f1987e8f9\"},{\"content\":{\"side\":\"RIGHT\"},\"type\":\"ConnectorPlacement.EquallySpacedRectSide\",\"uuid\":\"a3423ff2-a1bd-4263-8320-fe535760aa80\"},{\"content\":{\"connectorIds\":[\"In1\"],\"side\":\"TOP\"},\"type\":\"ConnectorPlacement.EquallySpacedRectSide\",\"uuid\":\"1adafbb7-f7c4-42e4-8eab-5e40445049e0\"}]},\"type\":\"ConnectorPlacement.EquallySpacedConnector\",\"uuid\":\"61c95f4c-4142-4f56-9fe1-ea528e3e26a5\"}],\"packageUris\":[\"http://schema.mathworks.com/mf0/Connector/R2020b\"],\"version\":\"1.0\"}"
  tag scope: r_est=global
  wires:
  Gain1/1 -> Gain3/1  "Rear Wheel Lateral Force (N)"
  [alpha_F] -> Gain/1, Mux/1  "Front Wheel Slip Angle (deg)"
  Gain4/1 -> To File/1, [r_est], Yaw Rate Error/1(r_est)  "Target Yaw Rate (deg/s)"
  Sum/1 -> Gain4/1  "Vehicle Yaw Moment (Nm)"
  Gain2/1 -> Sum/1  "Front Yaw Moment (Nm)"
  Gain/1 -> Gain2/1  "Front Wheel Lateral Force (N)"
  Gain3/1 -> Sum/2  "Rear Yaw Moment (Nm)"
  [alpha_R] -> Mux/2, Gain1/1  "Rear Wheel Slip Angle (deg)"
  Mux/1 -> Slip Angle Scope/1

== system cbuildv1p1/Control System/Driver Assists/Torque Vectoring/Throttle Pedal ==
  P_T : Inport
  Tmax : Inport  Port=2
  Product : Product
  CMD_T : Outport
  wires:
  P_T/1 -> Product/2  "Throttle Pedal Position (-)"
  Product/1 -> CMD_T/1  "Throttle Pedal Torque Command (Nm)"
  Tmax/1 -> Product/1  "Maximum Motor Torque (Nm)"

== system cbuildv1p1/Control System/Driver Assists/Traction Control/Slip Ratio Calculator ==
  Vx : Inport
  omega_RL : Inport  Port=2
  omega_RR : Inport  Port=3
  Constant : Constant
  Demux : Demux  Outputs=2
  Divide : Product  Inputs=*/
  Gain : Gain  Gain=1/60
  Gain1 : Gain  Gain=2*3.1415*R_e
  Minus : Sum  Inputs=+-
  Mux : Mux  Inputs=2
  Slip Ratio Scope : Scope
  kappa_RL : Outport
  kappa_RR : Outport  Port=2
  wires:
  omega_RL/1 -> Mux/1
  omega_RR/1 -> Mux/2
  Mux/1 -> Gain/1
  Gain/1 -> Gain1/1
  Vx/1 -> Divide/2  "Vehicle Velocity (m/s)"
  Demux/1 -> kappa_RL/1  "RL Slip Ratio (-)"
  Demux/2 -> kappa_RR/1  "RR Slip Ratio (-)"
  Divide/1 -> Minus/1
  Constant/1 -> Minus/2
  Minus/1 -> Slip Ratio Scope/1, Demux/1
  Gain1/1 -> Divide/1

== system cbuildv1p1/Control System/Driver Assists/Traction Control/Subsystem ==
  CMD_TV : Inport
  Enable : EnablePort
  Gain : Gain  Gain=TC_CUT
  CMD_TC : Outport
  wires:
  Gain/1 -> CMD_TC/1  "TC Torque Command (Nm)"
  CMD_TV/1 -> Gain/1  "TV Torque Command (Nm)"

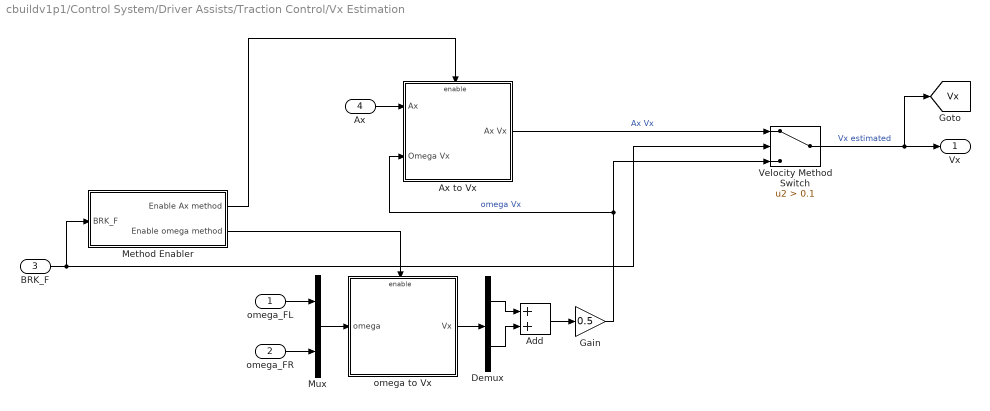
== system cbuildv1p1/Control System/Driver Assists/Traction Control/Vx Estimation ==
  omega_FL : Inport
  omega_FR : Inport  Port=2
  BRK_F : Inport  Port=3
  Ax : Inport  Port=4
  Add : Sum
  Ax to Vx : Subsystem
  Demux : Demux  Outputs=2
  Gain : Gain  Gain=0.5
  Method Enabler : Subsystem
  Mux : Mux  Inputs=2
  Velocity Method Switch : Switch  Criteria=u2 > Threshold  Threshold=0.1  SaturateOnIntegerOverflow=off  InputSameDT=off
  omega to Vx : Subsystem
  Vx : Outport
  tag scope: Vx=global
  wires:
  Mux/1 -> omega to Vx/1(omega)
  omega to Vx/1(Vx) -> Demux/1
  Demux/2 -> Add/2
  omega_FR/1 -> Mux/2
  omega_FL/1 -> Mux/1
  Demux/1 -> Add/1
  BRK_F/1 -> Velocity Method Switch/2, Method Enabler/1(BRK_F)
  Add/1 -> Gain/1
  Gain/1 -> Velocity Method Switch/3, Ax to Vx/2(Omega Vx)  "omega Vx"
  Velocity Method Switch/1 -> [Vx], Vx/1  "Vx estimated"
  Ax/1 -> Ax to Vx/1(Ax)
  Ax to Vx/1(Ax Vx) -> Velocity Method Switch/1  "Ax Vx"
  Method Enabler/2(Enable omega method) -> omega to Vx/Enable
  Method Enabler/1(Enable Ax method) -> Ax to Vx/Enable

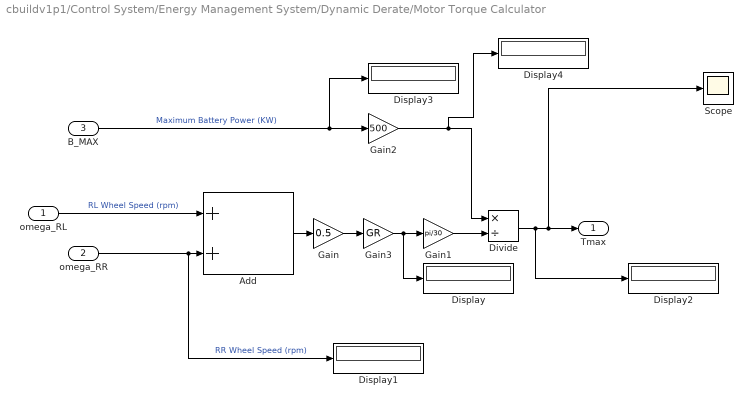
== system cbuildv1p1/Control System/Energy Management System/Dynamic Derate/Motor Torque Calculator ==
  omega_RL : Inport
  omega_RR : Inport  Port=2
  B_MAX : Inport  Port=3
  Add : Sum
  Display{,1..4} (5 alike) : Display
  Divide : Product  Inputs=*/
  Gain : Gain  Gain=0.5
  Gain1 : Gain  Gain=pi/30
  Gain2 : Gain  Gain=500
  Gain3 : Gain  Gain=GR
  Scope : Scope
  Tmax : Outport
  wires:
  omega_RR/1 -> Display1/1, Add/2  "RR Wheel Speed (rpm)"
  Add/1 -> Gain/1
  omega_RL/1 -> Add/1  "RL Wheel Speed (rpm)"
  Gain/1 -> Gain3/1
  Gain1/1 -> Divide/2
  B_MAX/1 -> Display3/1, Gain2/1  "Maximum Battery Power (KW)"
  Divide/1 -> Display2/1, Scope/1, Tmax/1
  Gain2/1 -> Display4/1, Divide/1
  Gain3/1 -> Display/1, Gain1/1

== system cbuildv1p1/Battery Thermal Model/Battery Cells/Battery Heat Generation/Current Estimator/Power Estimator ==
  Add : Sum
  Gain : Gain  Gain=rpm_to_radpers
  Gain2 : Gain  Gain=rpm_to_radpers
  Product : Product
  Product1 : Product
  Scope : Scope
  Motor Power (W) : Outport
  wires:
  [omega_RL] -> Gain/1
  [CMD_RL] -> Product/1
  Gain/1 -> Product/2
  Gain2/1 -> Product1/2
  [CMD_RR] -> Product1/1
  [omega_RR] -> Gain2/1
  Product/1 -> Scope/1, Add/1  "Left Motor Power (W)"
  Product1/1 -> Add/2  "Right Motor Power (W)"
  Add/1 -> Motor Power (W)/1  "Motor Power (W)"

== system cbuildv1p1/Control System/Driver Assists/Torque Vectoring/Target Yaw Rate Estimator/Slip Angle Estimator ==
  note: \arctan\left(\frac{a}{R}\right)
  Front : Subsystem
  Rear : Subsystem

== system cbuildv1p1/Control System/Driver Assists/Torque Vectoring/Target Yaw Rate Estimator/Yaw Rate Error ==
  r_est : Inport
  Mux : Mux  Inputs=2
  Sum : Sum  Inputs=|+-
  To File : ToFile  Filename=yawrate
  To File1 : ToFile  Filename=yawrateerror
  Yaw Rate Error Scope : Scope
  Yaw Rate Scope : Scope
  wires:
  r_est/1 -> Mux/1, Sum/1  "Target Yaw Rate (deg/s)"
  [r] -> Mux/2, To File/1, Sum/2  "Yaw Rate (deg/s)"
  Sum/1 -> To File1/1, Yaw Rate Error Scope/1  "Yaw Rate Error (deg/s)"
  Mux/1 -> Yaw Rate Scope/1

== system cbuildv1p1/Control System/Driver Assists/Traction Control/Vx Estimation/Ax to Vx ==
  Ax : Inport
  Omega Vx : Inport  Port=2
  Enable : EnablePort
  Integrator : Integrator
  Plus : Sum
  to m/s^2 : Gain  Gain=g
  Ax Vx : Outport
  wires:
  Ax/1 -> to m/s^2/1
  Integrator/1 -> Plus/2
  Omega Vx/1 -> Plus/1
  Plus/1 -> Ax Vx/1
  to m/s^2/1 -> Integrator/1

== system cbuildv1p1/Control System/Driver Assists/Traction Control/Vx Estimation/Method Enabler ==
  BRK_F : Inport
  Constant : Constant  Value=0
  Constant1 : Constant
  Constant2 : Constant  Value=0
  Constant3 : Constant
  Switch : Switch  Criteria=u2 > Threshold  Threshold=0.1  SaturateOnIntegerOverflow=off  InputSameDT=off
  Switch1 : Switch  Criteria=u2 > Threshold  SaturateOnIntegerOverflow=off  InputSameDT=off
  Enable Ax method : Outport
  Enable omega method : Outport  Port=2
  wires:
  Constant1/1 -> Switch/3
  Constant/1 -> Switch/1
  BRK_F/1 -> Switch/2
  Constant2/1 -> Switch1/1
  Constant3/1 -> Switch1/3
  Switch1/1 -> Enable Ax method/1
  Switch/1 -> Enable omega method/1, Switch1/2

== system cbuildv1p1/Control System/Driver Assists/Traction Control/Vx Estimation/omega to Vx ==
  omega : Inport
  Enable : EnablePort
  Gain : Gain  Gain=R_e
  Gain1 : Gain  Gain=rpm_to_radpers
  Vx : Outport
  wires:
  omega/1 -> Gain1/1
  Gain/1 -> Vx/1
  Gain1/1 -> Gain/1

== system cbuildv1p1/Control System/Driver Assists/Torque Vectoring/Target Yaw Rate Estimator/Slip Angle Estimator/Front ==
  Atan : Trigonometry  Operator=atan
  Constant : Constant  Value=a
  Divide : Product  Inputs=*/
  Divide1 : Product  Inputs=*/
  Gain : Gain  Gain=c_factor
  Gain1 : Gain  Gain=rackdisp_to_steerangle
  Gain2 : Gain  Gain=1/3.6
  Gain3 : Gain  Gain=g
  Square : Math  Operator=square
  Sum : Sum  Inputs=|+-
  tag scope: alpha_F=global
  wires:
  [delta_SW] -> Gain/1  "Steering Wheel Angle (deg)"
  Gain/1 -> Gain1/1  "Rack Displacement (mm)"
  Gain1/1 -> Sum/2  "Front Wheel Steering Angle (deg)"
  [Vx] -> Gain2/1  "Vehicle Velocity (kph)"
  Gain2/1 -> Square/1  "Vehicle Velocity (m/s)"
  Square/1 -> Divide/1
  [Ay] -> Gain3/1  "Lateral Acceleration (G)"
  Gain3/1 -> Divide/2  "Lateral Acceleration (m/s^2)"
  Divide/1 -> Divide1/2  "Turning Radius (m)"
  Constant/1 -> Divide1/1  "CG to Front Wheel Distance (m)"
  Atan/1 -> Sum/1  "Slip Angle w/o Steering (deg)"
  Divide1/1 -> Atan/1
  Sum/1 -> [alpha_F]  "Front Wheel Slip Angle (deg)"

== system cbuildv1p1/Control System/Driver Assists/Torque Vectoring/Target Yaw Rate Estimator/Slip Angle Estimator/Rear ==
  Atan : Trigonometry  Operator=atan
  Constant : Constant  Value=l-a
  Divide : Product  Inputs=*/
  Divide1 : Product  Inputs=*/
  Gain2 : Gain  Gain=1/3.6
  Gain3 : Gain  Gain=g
  Square : Math  Operator=square
  tag scope: alpha_R=global
  wires:
  Divide/1 -> Divide1/2  "Turning Radius (m)"
  [Ay] -> Gain3/1  "Lateral Acceleration (G)"
  Atan/1 -> [alpha_R]  "Rear Wheel Slip Angle (deg)"
  Gain3/1 -> Divide/2  "Lateral Acceleration (m/s^2)"
  [Vx] -> Gain2/1  "Vehicle Velocity (kph)"
  Square/1 -> Divide/1
  Constant/1 -> Divide1/1  "CG to Rear Wheel Distance (m)"
  Gain2/1 -> Square/1  "Vehicle Velocity (m/s)"
  Divide1/1 -> Atan/1
